simulink model "model_1D"  (R2021b)
settings: Solver=VariableStepAuto  StartTime=0.0  StopTime=discretization_time  RelTol=1e-3
values from neighbouring files (symbols this model uses):
  state = current_state+[0.5*time_step^2*input+current_state(2)*time_step,time_step*input]    [Model_1D.m]    (also in Model_der_1D.m = [1,time_step;0,1]; Model_der_2D.m = [1,0,-sin(current_state(3))*0.5*(current_state(5)+current_st; Model_obs_1D.m = [1,0;0,1]; Model_obs_2D.m = [1,0,0,0,0;0,1,0,0,0;0,0,1,0,0;0,0,0,1,0;0,0,0,0,1])
settings Model: Creator=filip  LastModifiedBy=filip

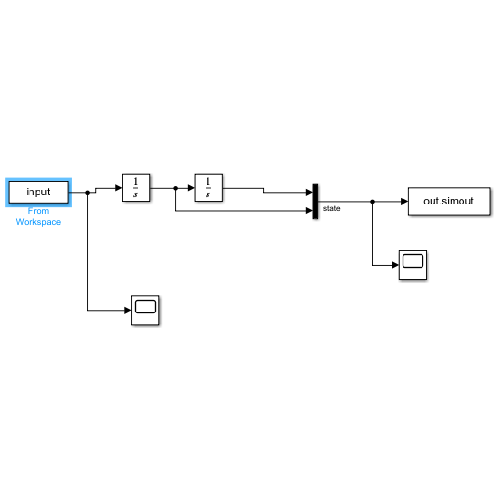
[thumbnail: Simulink's stored preview of the top-level diagram]
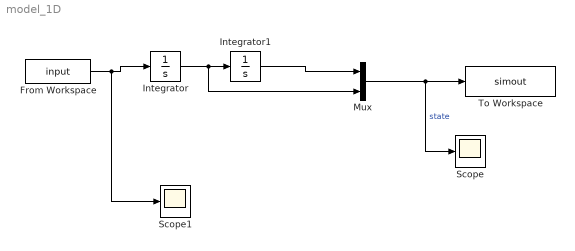
== system model_1D ==
  From Workspace : FromWorkspace  VariableName=input
  Integrator : Integrator  InitialCondition=state(2)
  Integrator1 : Integrator  InitialCondition=state(1)
  Mux : Mux  Inputs=2
  Scope : Scope
  Scope1 : Scope
  To Workspace : ToWorkspace  VariableName=simout  SaveFormat=Timeseries  SampleTime=-1
  wires:
  Integrator/1 -> Mux/2, Integrator1/1
  From Workspace/1 -> Scope1/1, Integrator/1
  Integrator1/1 -> Mux/1
  Mux/1 -> Scope/1, To Workspace/1  "state"
